simulink model "Lab6"  (R2015a)
settings: Solver=ode45  StartTime=0.0  StopTime=200  RelTol=1e-3
values from neighbouring files (symbols this model uses):
  K = 15*K/100    [mass_spring.m]
  L = 1    [RLC.m]
  R = 10    [RLC.m]
undefined symbols (not defined in the file or in its folder): b, J
libraries: elec_lib x1
settings Model: Creator=Bilal  LastModifiedBy=Bilal

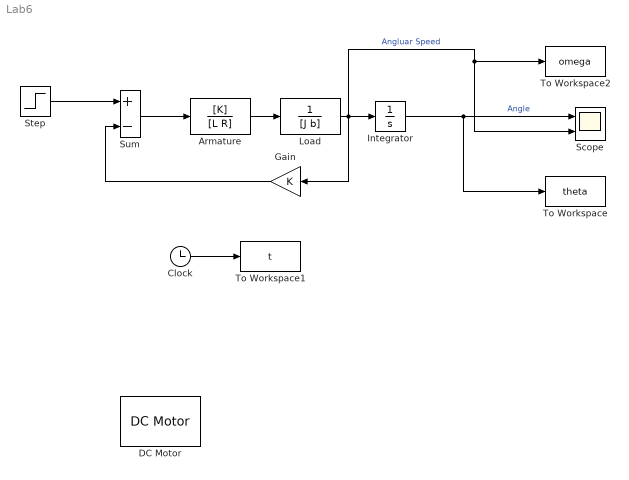
== system Lab6 ==
  Armature : TransferFcn  Numerator=[K]  Denominator=[L R]
  Clock : Clock
  DC Motor : elec_lib/Actuators & Drivers/Rotational Actuators/DC Motor  parameterization=1  Ra=3.9 Ohm  La=1.2e-5 H  emf_or_torque=1  Kv=7.2e-5 V/rpm  Ki=6.876e-4 N*m/A  T_stall=2.4e-4 N*m  w_max=1.91e+4 rpm  w_rated=1.5e+4 rpm  P_rated=0.08 W  V_rated=1.5 V  J=0.01 g*cm^2  lam_param=1  lam=0 N*m/(rad/s)  i_noload=0 A  V_i_noload=1.5 V  speed0=0 rpm  alpha=0.00393 1/K  Tmeas=25 C  thermal_mass=100 J/K  initial_temperature=25 C
  Gain : Gain  Gain=K
  Integrator : Integrator
  Load : TransferFcn  Denominator=[J b]
  "Scope " : Scope  NumInputPorts=2
      settings: ShowLegends=on  TimeRange=80  YMin=-5~0.5528169014084519  YMax=5~4.552816901408452
  Step : Step  SampleTime=0
  Sum : Sum  Inputs=+-
  To Workspace : ToWorkspace  VariableName=theta  SampleTime=-1
      settings: Save2DSignal=2-D array (concatenate along first dimension)
  To Workspace1 : ToWorkspace  VariableName=t  SampleTime=-1
      settings: Save2DSignal=2-D array (concatenate along first dimension)
  To Workspace2 : ToWorkspace  VariableName=omega  SampleTime=-1
      settings: Save2DSignal=2-D array (concatenate along first dimension)
  wires:
  Step/1 -> Sum/1
  Integrator/1 -> To Workspace/1, "Scope "/1  "Angle"
  Gain/1 -> Sum/2
  Sum/1 -> Armature/1
  Clock/1 -> To Workspace1/1
  Load/1 -> Gain/1, To Workspace2/1, "Scope "/2, Integrator/1  "Angluar Speed"
  Armature/1 -> Load/1
